simulink model "PLC_Peakshaving"  (R2023a)
settings: Solver=FixedStepDiscrete  StartTime=0.0  StopTime=90  FixedStep=Ts  RelTol=1e-3
values from neighbouring files (symbols this model uses):
  Ts_PLC = 0.001    [microgrid_system.sldd]
settings Model: DataDictionary=microgrid_system.sldd  SimulationMode=accelerator  Creator=jlesage  LastModifiedBy=steve.liu
settings SolverCC: AlgebraicLoopSolver=TrustRegion
settings OptimizationCC: ReuseModelBlockBuffer=off
settings DebuggingCC: UnconnectedInputMsg=warning  UnconnectedOutputMsg=warning  UnconnectedLineMsg=warning
settings ModelReferenceCC: EnableRefExpFcnMdlSchedulingChecks=on
settings RTWCC: DLArmComputeVersion=19.05
settings ConfigComp: PLC_TargetIDE=tiaportal_double  PLC_MultiTBSigbuilderTimeRange=off  PLC_FoldFBCallOutputVar=off  PLC_RemoveUnusedSSMethodCallArguments=off  PLC_UseCallOutputArgSyntax=off  PLC_EnableUnsignedAndDoubleTypes=off  PLC_EnableUDTSplitting=off  PLC_MaxFieldsInUDT=500  PLC_InlineEnumCastFunction=off

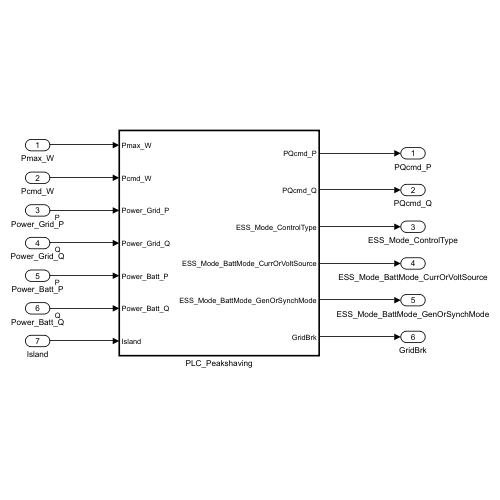
[thumbnail: Simulink's stored preview of the top-level diagram]
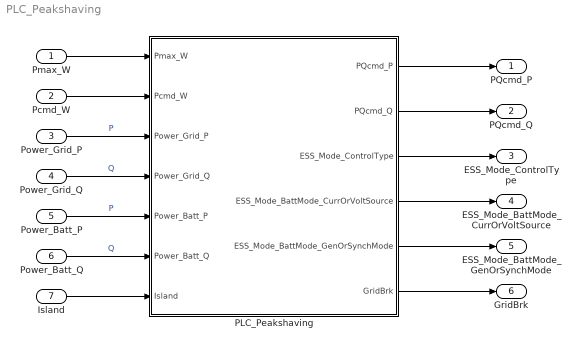
== system PLC_Peakshaving ==
  Pmax_W : Inport
  Pcmd_W : Inport  Port=2
  Power_Grid_P : Inport  Port=3
  Power_Grid_Q : Inport  Port=4
  Power_Batt_P : Inport  Port=5
  Power_Batt_Q : Inport  Port=6
  Island : Inport  Port=7
  PLC_Peakshaving : Subsystem  TreatAsAtomicUnit=on
  PQcmd_P : Outport  SampleTime=Ts_PLC
  PQcmd_Q : Outport  Port=2  SampleTime=Ts_PLC
  ESS_Mode_ControlType : Outport  Port=3  SampleTime=Ts_PLC
  ESS_Mode_BattMode_CurrOrVoltSource : Outport  Port=4  SampleTime=Ts_PLC
  ESS_Mode_BattMode_GenOrSynchMode : Outport  Port=5  SampleTime=Ts_PLC
  GridBrk : Outport  Port=6  SampleTime=Ts_PLC
  wires:
  PLC_Peakshaving/1(PQcmd_P) -> PQcmd_P/1
  PLC_Peakshaving/3(ESS_Mode_ControlType) -> ESS_Mode_ControlType/1
  PLC_Peakshaving/4(ESS_Mode_BattMode_CurrOrVoltSource) -> ESS_Mode_BattMode_CurrOrVoltSource/1
  PLC_Peakshaving/5(ESS_Mode_BattMode_GenOrSynchMode) -> ESS_Mode_BattMode_GenOrSynchMode/1
  PLC_Peakshaving/6(GridBrk) -> GridBrk/1
  PLC_Peakshaving/2(PQcmd_Q) -> PQcmd_Q/1
  Power_Batt_Q/1 -> PLC_Peakshaving/6(Power_Batt_Q)  "Q"
  Island/1 -> PLC_Peakshaving/7(Island)
  Power_Batt_P/1 -> PLC_Peakshaving/5(Power_Batt_P)  "P"
  Power_Grid_Q/1 -> PLC_Peakshaving/4(Power_Grid_Q)  "Q"
  Power_Grid_P/1 -> PLC_Peakshaving/3(Power_Grid_P)  "P"
  Pcmd_W/1 -> PLC_Peakshaving/2(Pcmd_W)
  Pmax_W/1 -> PLC_Peakshaving/1(Pmax_W)

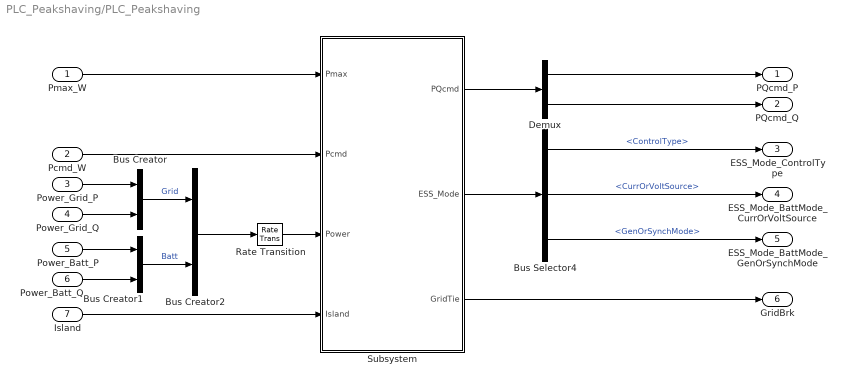
== system PLC_Peakshaving/PLC_Peakshaving ==
  Pmax_W : Inport
  Pcmd_W : Inport  Port=2
  Power_Grid_P : Inport  Port=3
  Power_Grid_Q : Inport  Port=4
  Power_Batt_P : Inport  Port=5
  Power_Batt_Q : Inport  Port=6
  Island : Inport  Port=7
  Bus Creator : BusCreator  Inputs=2
  Bus Creator1 : BusCreator  Inputs=2
  Bus Creator2 : BusCreator  Inputs=2
  Bus Selector4 : BusSelector  OutputSignals=ControlType,Bus_Batt_Mode.CurrOrVoltSource,Bus_Batt_Mode.GenOrSynchMode
  Demux : Demux  Outputs=2
  Rate Transition : RateTransition  OutPortSampleTime=Ts_PLC
  Subsystem : Subsystem  TreatAsAtomicUnit=on
  PQcmd_P : Outport  SampleTime=Ts_PLC
  PQcmd_Q : Outport  Port=2  SampleTime=Ts_PLC
  ESS_Mode_ControlType : Outport  Port=3  SampleTime=Ts_PLC
  ESS_Mode_BattMode_CurrOrVoltSource : Outport  Port=4  SampleTime=Ts_PLC
  ESS_Mode_BattMode_GenOrSynchMode : Outport  Port=5  SampleTime=Ts_PLC
  GridBrk : Outport  Port=6  SampleTime=Ts_PLC
  wires:
  Island/1 -> Subsystem/4(Island)
  Subsystem/1(PQcmd) -> Demux/1
  Bus Selector4/3 -> ESS_Mode_BattMode_GenOrSynchMode/1  "<GenOrSynchMode>"
  Pmax_W/1 -> Subsystem/1(Pmax)
  Subsystem/2(ESS_Mode) -> Bus Selector4/1
  Bus Creator1/1 -> Bus Creator2/2  "Batt"
  Power_Batt_Q/1 -> Bus Creator1/2
  Subsystem/3(GridTie) -> GridBrk/1
  Power_Grid_Q/1 -> Bus Creator/2
  Demux/2 -> PQcmd_Q/1
  Bus Creator2/1 -> Rate Transition/1
  Demux/1 -> PQcmd_P/1
  Bus Creator/1 -> Bus Creator2/1  "Grid"
  Bus Selector4/2 -> ESS_Mode_BattMode_CurrOrVoltSource/1  "<CurrOrVoltSource>"
  Power_Batt_P/1 -> Bus Creator1/1
  Power_Grid_P/1 -> Bus Creator/1
  Bus Selector4/1 -> ESS_Mode_ControlType/1  "<ControlType>"
  Rate Transition/1 -> Subsystem/3(Power)
  Pcmd_W/1 -> Subsystem/2(Pcmd)

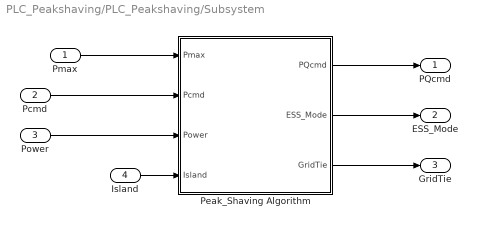
== system PLC_Peakshaving/PLC_Peakshaving/Subsystem ==
  Pmax : Inport
  Pcmd : Inport  Port=2
  Power : Inport  Port=3
  Island : Inport  Port=4
  Peak_Shaving Algorithm : Stateflow chart  TreatAsAtomicUnit=on  SystemSampleTime=Ts_PLC
  PQcmd : Outport
  ESS_Mode : Outport  Port=2
  GridTie : Outport  Port=3
  wires:
  Peak_Shaving Algorithm/1(PQcmd) -> PQcmd/1
  Pcmd/1 -> Peak_Shaving Algorithm/2(Pcmd)
  Pmax/1 -> Peak_Shaving Algorithm/1(Pmax)
  Peak_Shaving Algorithm/2(ESS_Mode) -> ESS_Mode/1
  Island/1 -> Peak_Shaving Algorithm/4(Island)
  Peak_Shaving Algorithm/3(GridTie) -> GridTie/1
  Power/1 -> Peak_Shaving Algorithm/3(Power)

== stateflow chart PLC_Peakshaving/Subsystem/Peak_Shaving Algorithm ==
  state ESS_Control [parallel]
    during:
    P_Excess = Power.Grid.P + Power.Batt.P + Pcmd - Pmax;
    P_Max = genMax - Power.Batt.P;
    settings: executionOrder=1
    state GridConnected
      entry,during:
      ESS_Mode.ControlType = 0; %PQ Mode
      ESS_Mode.Batt_Mode.CurrOrVoltSource = 0; %Current Source
      isIsland = 0;
      state PeakShaving
        state MaxLocalGeneration
          during:
          PQcmd = [P_Max;0];
        state LoadFollowing
          during:
          PQcmd = [P_Excess;0];
        (default) -> LoadFollowing
        MaxLocalGeneration -> LoadFollowing : [Power.Batt.P < 0.95*genMax]
        LoadFollowing -> MaxLocalGeneration : [Power.Batt.P > genMax]
      state Nominal
        entry,during:
        PQcmd = [Pcmd;0];
      Nominal -> PeakShaving : [Power.Grid.P + Pcmd ...
          |  > Pmax]
      PeakShaving -> Nominal : [Power.Batt.P < 0 ...
          | && after(1,sec)]
      (default) -> Nominal
    state PrepareToIsland
      entry,during:
      PQcmd = [Power.Grid.P + Power.Batt.P + Pcmd; 0];
    state Islanded
      during:
      ESS_Mode.Batt_Mode.CurrOrVoltSource = 1; %Voltage Source
      ESS_Mode.Batt_Mode.GenOrSynchMode = 0; % No synch
      ESS_Mode.ControlType = 2; %No Current Control
    state Synchronize
      entry,during:
      ESS_Mode.Batt_Mode.CurrOrVoltSource = 1; %Voltage Source
      ESS_Mode.Batt_Mode.GenOrSynchMode = 1; % Synchronize
    (default) -> GridConnected
    GridConnected -> PrepareToIsland : [Island == 1]
    ESS_Control.Synchronize -> GridConnected : Reconnect
    PrepareToIsland -> ESS_Control.Islanded : [Power.Grid.P < 100]{isIsland = 1;}
    ESS_Control.Islanded -> ESS_Control.Synchronize : Synchronize
  state GridBreakerLogic [parallel]
    settings: executionOrder=2
    state Islanded
      during:
      GridTie = 0;
    state GridTied
      entry,during:
      GridTie = 1;
    state Reconnect
      entry,during:
      GridTie = 1;
      isIsland = 0;
    state Synchronize
    (default) -> GridTied
    GridTied -> GridBreakerLogic.Islanded : [isIsland == 1]
    Reconnect -> GridTied : [after(1,sec)] {send(Reconnect,ESS_Control)}
    GridBreakerLogic.Islanded -> GridBreakerLogic.Synchronize : [after(1,sec) && Island == 0] {send(Synchronize,ESS_Control)}
    GridBreakerLogic.Synchronize -> Reconnect : [after(2,sec)]
  data: Pmax input; genMax parameter; Pcmd input; Power input Bus: PowerBus; PQcmd output; ESS_Mode output Bus: ESS_Mode =0; GridTie output; P_Excess local; P_Max local; Island input; isIsland local
  events: Reconnect local FUNCTION_CALL_EVENT; Synchronize local FUNCTION_CALL_EVENT
